simulink model "ECE675_HW3_Problem3_sim_b"  (R2025b)
settings: Solver=VariableStepAuto  StartTime=0.0  StopTime=10.0  RelTol=1e-3
values from neighbouring files (symbols this model uses):
  x0 = x_next    [ECE675_HW3.m]    (also in ECE675_HW3_v2.m = [pi/2; 0]; ECE675_HW3_v3.m = [pi/2; 0])
undefined symbols (not defined in the file or in its folder): Ad_lin, Bd_lin, Cd_lin, Dd_lin, ts
settings Model: Creator=iwant  LastModifiedBy=iwant

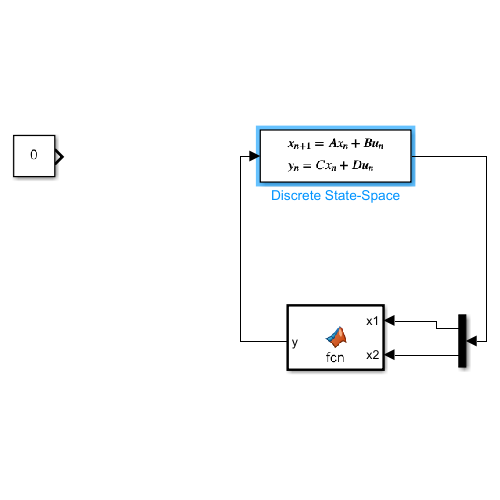
[thumbnail: Simulink's stored preview of the top-level diagram]
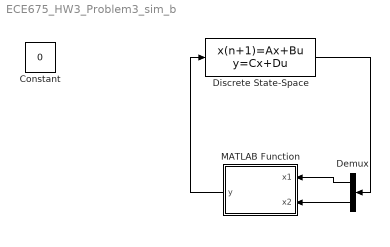
== system ECE675_HW3_Problem3_sim_b ==
  Constant : Constant  Value=0
  Demux : Demux  Outputs=2
  Discrete State-Space : DiscreteStateSpace  A=Ad_lin  B=Bd_lin  C=Cd_lin  D=Dd_lin  InitialCondition=x0  SampleTime=ts
  MATLAB Function : MATLAB Function  TreatAsAtomicUnit=on
  wires:
  Discrete State-Space/1 -> Demux/1
  MATLAB Function/1(y) -> Discrete State-Space/1
  Demux/1 -> MATLAB Function/1(x1)
  Demux/2 -> MATLAB Function/2(x2)

== matlab function ECE675_HW3_Problem3_sim_b/MATLAB Function ==
  data: x1 input; y output; x2 input
function y = fcn(x1, x2)
    x_state = [x1; x2];
y = GetOptimalInput(x_state);
